simulink model "11_1"  (R2018b)
settings: Solver=VariableStepAuto  StartTime=0.0  StopTime=5  MaxStep=0.01  RelTol=1e-3
InitFcn:
  | Gg = [0 1; -25 0];
  | Hg = [1 0];
  | 
  | G = [0 1; -25 0];
  | H = [1 0];
  | 
  | G_sh = [0 -(16/3)^2; 1 -32/3];
  | L_sh = [0; 1];
  | 
  | M_sh = sylv(-G_sh,G,L_sh.*H);
  | 
  | A = [0 1; 4 0];
  | B = [1; 1];
  | C = [3 0];
  | D = 3;
  | 
  | 
  | H = [1 1];
  | G = [-15 0; 0 -6];
  | 
  | syms m11 m12 m21 m22 k1 k2;
  | M = [m11 m12; m21 m22];
  | K = [k1 k2];
  | 
  | eqn1 = B*H == M*G - A*M;
  | eqn2 = K == -H*inv(M);
  | 
  | sol = solve([eqn1,eqn2], [m11, m12, m21, m22, k1, k2]);
  | m11Sol = double(sol.m11);
  | m12Sol = double(sol.m12);
  | m21Sol = double(sol.m21);
  | m22Sol = double(sol.m22);
  | k1Sol = double(sol.k1);
  | k2Sol = double(sol.k2);
  | 
  | Msol = [m11Sol m12Sol; m21Sol m22Sol];
  | K_sol = [k1Sol k2Sol];
  | 
  | 
  | 
  | 
  | 
  | G = [0 1; -25 0];
  | H = [1 0];
  | 
  | syms m11 m12 m21 m22 l1 l2;
  | M = [m11 m12; m21 m22];
  | L = [l1 l2];
  | 
  | eqn1 = B*L == M*G - (A-B*K_sol)*M;
  | eqn2 = H == (C-D*K_sol)*M + D*L;
  | 
  | sol = solve([eqn1,eqn2], [m11, m12, m21, m22, l1, l2]);
  | m11Sol = double(sol.m11);
  | m12Sol = double(sol.m12);
  | m21Sol = double(sol.m21);
  | m22Sol = double(sol.m22);
  | l1Sol = double(sol.l1);
  | l2Sol = double(sol.l2);
  | 
  | Msol = [m11Sol m12Sol; m21Sol m22Sol];
  | Lg = [l1Sol l2Sol];
settings Model: Creator=kekos  LastModifiedBy=kekos

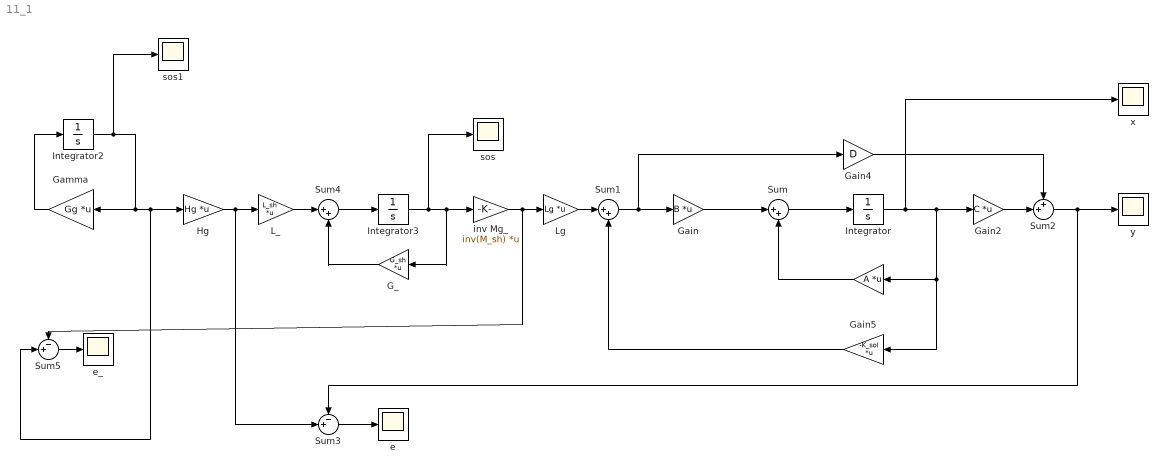
== system 11_1 ==
  " " : Gain  Gain=A  Multiplication=Matrix(K*u)
  " G_" : Gain  Gain=G_sh  Multiplication=Matrix(K*u)
  Gain : Gain  Gain=B  Multiplication=Matrix(K*u)
  Gain2 : Gain  Gain=C  Multiplication=Matrix(K*u)
  Gain4 : Gain  Gain=D
  Gain5 : Gain  Gain=-K_sol  Multiplication=Matrix(K*u)
  Gamma : Gain  Gain=Gg  Multiplication=Matrix(K*u)
  Hg : Gain  Gain=Hg  Multiplication=Matrix(K*u)
  Integrator : Integrator
  Integrator2 : Integrator  InitialCondition=[0.91; -2.08]
  Integrator3 : Integrator
  L_ : Gain  Gain=L_sh  Multiplication=Matrix(K*u)
  "Lg " : Gain  Gain=Lg  Multiplication=Matrix(K*u)
  Sum : Sum  Inputs=|++
  Sum1 : Sum  Inputs=|++
  Sum2 : Sum  Inputs=++|
  Sum3 : Sum  Inputs=-+|
  Sum4 : Sum  Inputs=|++
  Sum5 : Sum  Inputs=-+|
  e : Scope
  e_ : Scope
  inv Mg_ : Gain  Gain=inv(M_sh)  Multiplication=Matrix(K*u)
  sos : Scope
  sos1 : Scope
  x : Scope
  y : Scope
  wires:
  Gain2/1 -> Sum2/2
  Gain4/1 -> Sum2/1
  Gain/1 -> Sum/1
  Sum/1 -> Integrator/1
  Integrator/1 -> x/1, Gain2/1, " "/1, Gain5/1
  Sum2/1 -> Sum3/1, y/1
  " "/1 -> Sum/2
  Sum1/1 -> Gain4/1, Gain/1
  "Lg "/1 -> Sum1/1
  Gain5/1 -> Sum1/2
  Gamma/1 -> Integrator2/1
  L_/1 -> Sum4/1
  Sum4/1 -> Integrator3/1
  Integrator3/1 -> sos/1, " G_"/1, inv Mg_/1
  " G_"/1 -> Sum4/2
  Hg/1 -> L_/1, Sum3/2
  Sum3/1 -> e/1
  inv Mg_/1 -> Sum5/1, "Lg "/1
  Sum5/1 -> e_/1
  Integrator2/1 -> sos1/1, Sum5/2, Hg/1, Gamma/1
